simulink model "unicycle_differential_drive_excercise_R2018a"  (R2018a)
settings: Solver=VariableStepAuto  StartTime=0.0  StopTime=1.2  MaxStep=1e-3  RelTol=1e-3
libraries: simulink x1
settings Model: EnablePacing=on  PacingRate=0.450000  Creator=kjartan  LastModifiedBy=kjartan
settings DataIOCC: ReturnWorkspaceOutputs=on
settings DebuggingCC: SFMachineParentedDataDiag=error
settings SFSimCC: SimUseLocalCustomCode=on
settings RTWCC: RTWUseLocalCustomCode=on

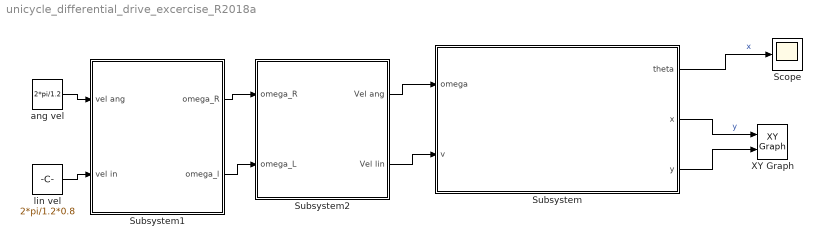
== system unicycle_differential_drive_excercise_R2018a ==
  Scope : Scope
  Subsystem : Subsystem
  Subsystem1 : Subsystem
  Subsystem2 : Subsystem
  XY Graph : simulink/Sinks/XY Graph  xmin=-1  xmax=1  ymin=-1  ymax=1  st=-1
  ang vel : Constant  Value=2*pi/1.2
  lin vel : Constant  Value=2*pi/1.2*0.8
  wires:
  Subsystem/2(x) -> XY Graph/1  "y"
  Subsystem/3(y) -> XY Graph/2
  Subsystem/1(theta) -> Scope/1  "x"
  ang vel/1 -> Subsystem1/1(vel ang)
  lin vel/1 -> Subsystem1/2(vel in)
  Subsystem1/1(omega_R) -> Subsystem2/1(omega_R)
  Subsystem1/2(omega_l) -> Subsystem2/2(omega_L)
  Subsystem2/1(Vel ang) -> Subsystem/1(omega)
  Subsystem2/2(Vel lin) -> Subsystem/2(v)

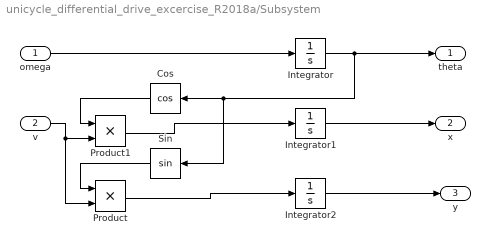
== system unicycle_differential_drive_excercise_R2018a/Subsystem ==
  omega : Inport
  v : Inport  Port=2
  Cos : Trigonometry  Operator=cos
  Integrator : Integrator  InitialCondition=pi/2
  Integrator1 : Integrator  InitialCondition=2
  Integrator2 : Integrator  InitialCondition=2
  Product : Product
  Product1 : Product
  Sin : Trigonometry
  theta : Outport
  x : Outport  Port=2
  y : Outport  Port=3
  wires:
  Integrator1/1 -> x/1
  v/1 -> Product1/2, Product/2
  Integrator/1 -> Sin/1, Cos/1, theta/1
  omega/1 -> Integrator/1
  Integrator2/1 -> y/1
  Product/1 -> Integrator2/1
  Sin/1 -> Product/1
  Product1/1 -> Integrator1/1
  Cos/1 -> Product1/1

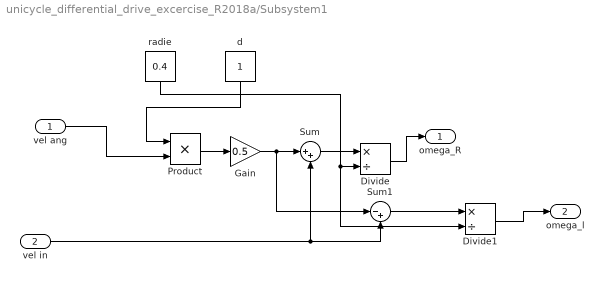
== system unicycle_differential_drive_excercise_R2018a/Subsystem1 ==
  vel ang : Inport
  vel in : Inport  Port=2
  Divide : Product  Inputs=*/
  Divide1 : Product  Inputs=*/
  Gain : Gain  Gain=0.5
  Product : Product
  Sum : Sum  Inputs=|++
  Sum1 : Sum  Inputs=|-+
  d : Constant
  radie : Constant  Value=0.4
  omega_R : Outport
  omega_l : Outport  Port=2
  wires:
  d/1 -> Product/1
  vel ang/1 -> Product/2
  Product/1 -> Gain/1
  Sum/1 -> Divide/1
  radie/1 -> Divide1/2, Divide/2
  Divide/1 -> omega_R/1
  vel in/1 -> Sum1/2, Sum/2
  Gain/1 -> Sum1/1, Sum/1
  Sum1/1 -> Divide1/1
  Divide1/1 -> omega_l/1

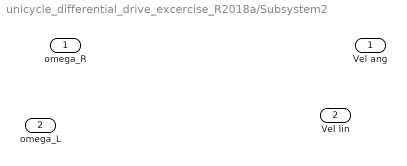
== system unicycle_differential_drive_excercise_R2018a/Subsystem2 ==
  omega_R : Inport
  omega_L : Inport  Port=2
  Vel ang : Outport
  Vel lin : Outport  Port=2
